simulink model "open_loop_2020a"  (R2020a)
settings: Solver=FixedStepAuto  StartTime=0.0  StopTime=10  FixedStep=1/100  RelTol=1e-3  AbsTol=1e-3
model workspace: external: MATLAB File params.m (data not in the file)
values from neighbouring files (symbols this model uses):
  A = subs(jacobian(f,x), [x; u], [zeros(12,1); init_u])    [check_state_space.m]    (also in genStateSpaceMat.m = double(subs(jacobian(f,x), [x; u], [zeros(12,1); init_u])))
  B = subs(jacobian(f,u), [x; u], [zeros(12,1); init_u])    [check_state_space.m]    (also in genStateSpaceMat.m = B.*MF.*180/pi)
  C = blkdiag(180/pi .* eye(6), eye(6))    [check_state_space.m]    (also in genStateSpaceMat.m)
  D = zeros(12,4)    [check_state_space.m]    (also in genStateSpaceMat.m)
undefined symbols (not defined in the file or in its folder): DiscIntNeverNeededParam, dt, g
libraries: nesl_utility x9
settings Model: Creator=Jocke  LastModifiedBy=parke
settings SolverCC: AutoScaleAbsTol=off
settings DataIOCC: ReturnWorkspaceOutputs=off
settings DebuggingCC: ArithmeticOperatorsInVariantConditions=warning
settings SFSimCC: SimUseLocalCustomCode=off  CustomCodeUndefinedFunction=UseInterfaceOnly
settings RTWCC: RTWUseLocalCustomCode=off
settings CodeAppCC: StateflowObjectComments=on
settings SimscapeCC: SimscapeNormalizeSystem=off  SimscapeLogType=all  SimscapeLogDataHistory=10000

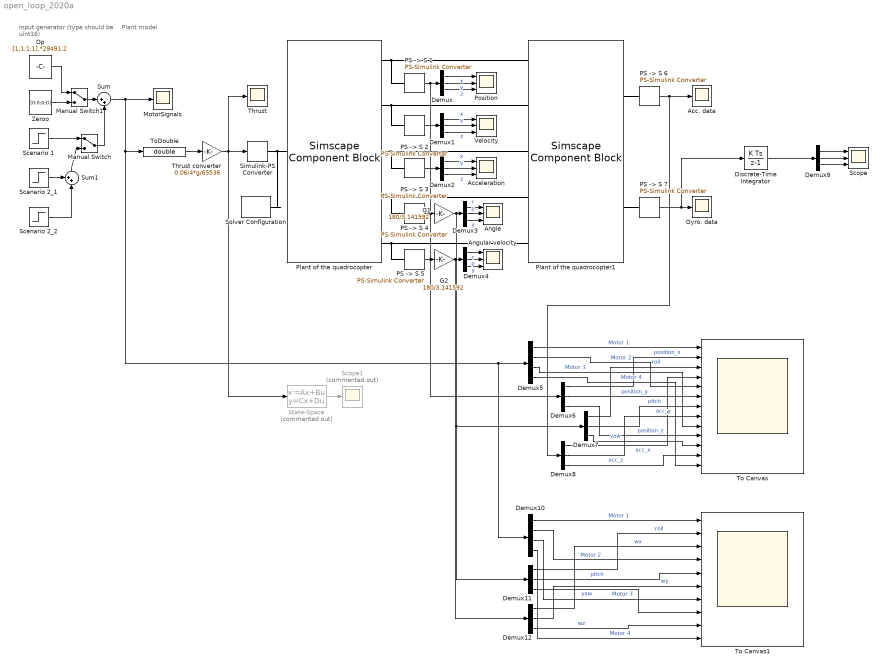
== system open_loop_2020a ==
  note: Input generator
      | (type should be uint16)
  note: Plant model
  Acc. data : Scope
  Acceleration : Scope  NumInputPorts=3
  Angle : Scope  NumInputPorts=3
  Angular velocity : Scope  NumInputPorts=3
  Demux{,1..4,6..9,11..12} (11 alike) : Demux  Outputs=3
  Demux10 : Demux
  Demux5 : Demux
  Discrete-Time Integrator : DiscreteIntegrator  SampleTime=-1  ICPrevOutput=DiscIntNeverNeededParam  ICPrevScaledInput=DiscIntNeverNeededParam
  G1 : Gain  Gain=180/3.141592
  G2 : Gain  Gain=180/3.141592
  Gyro. data : Scope
  Manual Switch : ManualSwitch
  Manual Switch1 : ManualSwitch
  MotorSignals : Scope
  Op : Constant  Value=[1;1;1;1].*29491.2  VectorParams1D=off  OutDataTypeStr=uint16
  PS -> S {1..7} (7 alike) : nesl_utility/PS-Simulink Converter  PhysicalDomain=network_engine_domain  SubClassName=ps_output  LeftPortType=input  RightPortType=output  PseudoPeriodic=off  Frequencies=[]  Unit=1  AffineConversion=off
  Plant of the quadrocopter : SimscapeComponentBlock  SourceFile=plant  ComponentPath=plant  ComponentVariants="[\"plant\"]"  ComponentVariantNames="[\"plant\"]"  ClassName=plant  SchemaVersion=1  m=0.027 kg  g=9.81 m/s^2  d=0.046 m  k=2.5383e-11 m  b=1.9796e-9  F=0.1 N/(m/s)
      settings: CopyFcn=simscape.engine.sli.internal.componentblockcallback(gcbh,'COPY')  PreCopyFcn=simscape.engine.sli.internal.componentblockcallback(gcbh,'PRECOPY')  PreDeleteFcn=simscape.engine.sli.internal.componentblockcallback(gcbh,'PREDELETE')  InternalSimscapePortConfiguration="{\"Bottom\":[],\"Left\":[{\"id\":\"ctrl\",\"label\":\"Thrust\",\"type\":\"input\"}],\"Right\":[{\"id\":\"pos\",\"label\":\"Position\",\"type\":\"output\"},{\"id\":\"v\",\"label\":\"Velocity\",\"type\":\"output\"},{\"id\":\"a\",\"label\":\"Acceleration\",\"type\":\"output\"},{\"id\":\"angle\",\"label\":\"Angle\",\"type\":\"output\"},{\"id\":\"w\",\"label\":\"Angular velocity\",\"type\":\"output\"}],\"Top\":[]}"
      mask Type: Plant of quadrocopter
  Plant of the quadrocopter1 : SimscapeComponentBlock  SourceFile=sensors1  ComponentPath=sensors1  ComponentVariants="[\"sensors1\"]"  ComponentVariantNames="[\"sensors1\"]"  ClassName=sensors1  SchemaVersion=1  m=0.027 kg  g=9.81 m/s^2  d=0.046 m  k=1e-9  b=2.75e-11  F=0.1 N/(m/s)
      settings: CopyFcn=simscape.engine.sli.internal.componentblockcallback(gcbh,'COPY')  PreCopyFcn=simscape.engine.sli.internal.componentblockcallback(gcbh,'PRECOPY')  PreDeleteFcn=simscape.engine.sli.internal.componentblockcallback(gcbh,'PREDELETE')  InternalSimscapePortConfiguration="{\"Bottom\":[],\"Left\":[{\"id\":\"pos\",\"label\":\"Position\",\"type\":\"input\"},{\"id\":\"v\",\"label\":\"Velocity\",\"type\":\"input\"},{\"id\":\"a\",\"label\":\"Acceleration\",\"type\":\"input\"},{\"id\":\"angle\",\"label\":\"Angle\",\"type\":\"input\"},{\"id\":\"w\",\"label\":\"Angular velocity\",\"type\":\"input\"}],\"Right\":[{\"id\":\"acc\",\"label\":\"Accelerometer\",\"type\":\"output\"},{\"id\":\"gyro\",\"label\":\"Gyroscope\",\"type\":\"output\"}],\"Top\":[]}"
      mask Type: Plant of quadrocopter
  Position : Scope  NumInputPorts=3
  Scenario 1 : Step  Time=4  Before=[0;0;0;0]  After=[0;10;10;0]  SampleTime=dt
  Scenario 2_1 : Step  Time=4  Before=[0;0;0;0]  After=[10;0;0;0]  SampleTime=dt
  Scenario 2_2 : Step  Time=6  Before=[0;0;0;0]  After=[0;0;20;0]  SampleTime=dt
  Scope : Scope  NumInputPorts=3
  Scope1 : Scope  Commented=on
  Simulink-PS Converter : nesl_utility/Simulink-PS Converter  PhysicalDomain=network_engine_domain  SubClassName=ps_input  LeftPortType=input  RightPortType=output  PseudoPeriodic=off  Frequencies=[]  NoiseDistribution=none  NoiseParameters=[]  Unit=1  AffineConversion=off  FilteringAndDerivatives=zero  SimscapeFilterOrder=1  InputFilterTimeConstant=0.001  UdotUserProvided=1
  Solver Configuration : nesl_utility/Solver Configuration  PhysicalDomain=network_engine_domain  SubClassName=solver  LeftPortType=input  RightPortType=generic  Tones=[]  Harmonics=[]  SimulateNoise=off  Profile=off  UseLocalSampling=off  EnableSwitchedLinearOptims=on  FrequencyDomain=off  UseCCode=off  RelTol=0.001  AbsTol=1e-06  MinStep=1e-09  ToWorkspace=off  RevertToSquareIcSolve=off  NumHomotopyIterations=100  PhasorMode=off  PhasorModeNumHarmonics=1  DoDC=off  ResidualTolerance=1e-09  UseLocalSolver=off  LocalSolverChoice=NE_BACKWARD_EULER_ADVANCER  LocalSolverSampleTime=0.001  DoFixedCost=off  MaxNonlinIter=3  MaxModeIter=2  LinearAlgebra=Sparse  EquationFormulation=NE_TIME_EF  DelaysMemoryBudget=1024  AutomaticFiltering=on  FilteringTimeConstant=0.001  PartitionStorageMethod=AS_NEEDED  PartitionMemoryBudget=1024  PartitionMethod=FAST
  State-Space : StateSpace  Commented=on  A=A  B=B  C=C  D=D  InitialCondition=0
  Sum : Sum  Inputs=|++
  Sum1 : Sum  Inputs=++|
  Thrust : Scope
  Thrust converter : Gain  Gain=0.06/4*g/65536
  To Canvas : Scope  NumInputPorts=13
  To Canvas1 : Scope  NumInputPorts=10
  ToDouble : DataTypeConversion  OutDataTypeStr=double  RndMeth=Round  SaturateOnIntegerOverflow=on
  Velocity : Scope  NumInputPorts=3
  Zeroo : Constant  Value=[0;0;0;0]  VectorParams1D=off  OutDataTypeStr=uint16
  wires:
  "PS -> S 7"/1 -> Discrete-Time Integrator/1, Gyro. data/1
  "PS -> S 6"/1 -> Demux8/1, Acc. data/1
  ToDouble/1 -> Thrust converter/1
  Thrust converter/1 -> State-Space/1, Simulink-PS Converter/1, Thrust/1
  "PS -> S 1"/1 -> Demux6/1, Demux/1
  "PS -> S 5"/1 -> G2/1
  "PS -> S 4"/1 -> G1/1
  "PS -> S 3"/1 -> Demux2/1
  "PS -> S 2"/1 -> Demux1/1
  Sum/1 -> MotorSignals/1, Demux10/1, Demux5/1, ToDouble/1
  Demux/1 -> Position/1  "x"
  Demux/2 -> Position/2  "y"
  Demux/3 -> Position/3  "z"
  Demux1/1 -> Velocity/1  "x"
  Demux1/2 -> Velocity/2  "y"
  Demux1/3 -> Velocity/3  "z"
  Demux2/1 -> Acceleration/1  "x"
  Demux2/2 -> Acceleration/2  "y"
  Demux2/3 -> Acceleration/3  "z"
  G1/1 -> Demux11/1, Demux7/1, Demux3/1
  Demux3/2 -> Angle/2  "p"
  Demux3/1 -> Angle/1  "r"
  Demux3/3 -> Angle/3  "y"
  G2/1 -> Demux12/1, Demux4/1
  Demux4/1 -> Angular velocity/1  "r"
  Demux4/2 -> Angular velocity/2  "p"
  Demux4/3 -> Angular velocity/3  "y"
  Scenario 1/1 -> Manual Switch/1
  Scenario 2_1/1 -> Sum1/1
  Sum1/1 -> Manual Switch/2
  Manual Switch1/1 -> Sum/1
  Op/1 -> Manual Switch1/1
  Zeroo/1 -> Manual Switch1/2
  Scenario 2_2/1 -> Sum1/2
  Demux5/1 -> To Canvas/1  "Motor 1"
  Demux6/1 -> To Canvas/2  "position_x"
  Demux7/1 -> To Canvas/3  "roll"
  Demux8/1 -> To Canvas/4  "acc_x"
  Demux5/2 -> To Canvas/5  "Motor 2"
  Demux6/2 -> To Canvas/6  "position_y"
  Demux7/2 -> To Canvas/7  "pitch"
  Demux8/2 -> To Canvas/8  "acc_y"
  Demux5/3 -> To Canvas/9  "Motor 3"
  Demux6/3 -> To Canvas/10  "position_z"
  Demux7/3 -> To Canvas/11  "yaw"
  Demux8/3 -> To Canvas/12  "acc_z"
  Demux5/4 -> To Canvas/13  "Motor 4"
  Demux9/1 -> Scope/1
  Demux9/2 -> Scope/2
  Demux9/3 -> Scope/3
  Discrete-Time Integrator/1 -> Demux9/1
  State-Space/1 -> Scope1/1
  Demux10/1 -> To Canvas1/1  "Motor 1"
  Demux11/1 -> To Canvas1/2  "roll"
  Demux12/1 -> To Canvas1/3  "wx"
  Demux10/2 -> To Canvas1/4  "Motor 2"
  Demux11/2 -> To Canvas1/5  "pitch"
  Demux12/2 -> To Canvas1/6  "wy"
  Demux10/3 -> To Canvas1/7  "Motor 3"
  Demux11/3 -> To Canvas1/8  "yaw"
  Demux12/3 -> To Canvas1/9  "wz"
  Demux10/4 -> To Canvas1/10  "Motor 4"
  Manual Switch/1 -> Sum/2
  connections:
  Plant of the quadrocopter/LConn1 -- Solver Configuration/RConn1 -- Simulink-PS Converter/RConn1
  Plant of the quadrocopter/RConn1 -- Plant of the quadrocopter1/LConn1 -- "PS -> S 1"/LConn1
  Plant of the quadrocopter/RConn2 -- Plant of the quadrocopter1/LConn2 -- "PS -> S 2"/LConn1
  Plant of the quadrocopter/RConn3 -- Plant of the quadrocopter1/LConn3 -- "PS -> S 3"/LConn1
  Plant of the quadrocopter/RConn4 -- Plant of the quadrocopter1/LConn4 -- "PS -> S 4"/LConn1
  Plant of the quadrocopter/RConn5 -- Plant of the quadrocopter1/LConn5 -- "PS -> S 5"/LConn1
  Plant of the quadrocopter1/RConn1 -- "PS -> S 6"/LConn1
  Plant of the quadrocopter1/RConn2 -- "PS -> S 7"/LConn1
